simulink model "LAB1schmN2"  (R2016a)
settings: Solver=VariableStepAuto  StartTime=0.0  StopTime=40  RelTol=1e-3
settings Model: Creator=Григорий  LastModifiedBy=Григорий

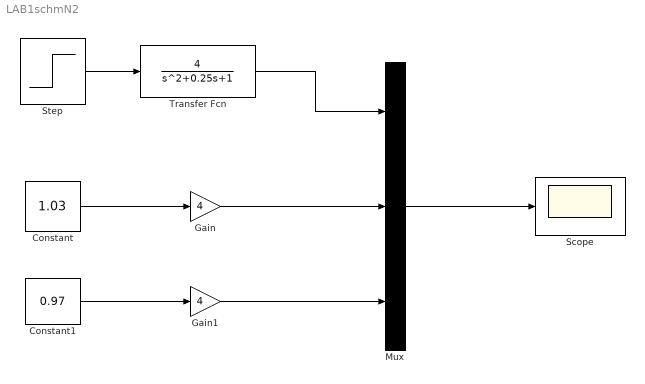
== system LAB1schmN2 ==
  Constant : Constant  Value=1.03
  Constant1 : Constant  Value=0.97
  Gain : Gain  Gain=4
  Gain1 : Gain  Gain=4
  Mux : Mux  Inputs=3
  Scope : Scope
  Step : Step  SampleTime=0
  Transfer Fcn : TransferFcn  Numerator=[4]  Denominator=[1 0.25 1]
  wires:
  Step/1 -> Transfer Fcn/1
  Mux/1 -> Scope/1
  Transfer Fcn/1 -> Mux/1
  Constant/1 -> Gain/1
  Gain/1 -> Mux/2
  Constant1/1 -> Gain1/1
  Gain1/1 -> Mux/3
